simulink model "Controle_controle"  (R2015a)
settings: Solver=ode45  StartTime=0.0  StopTime=Tsim  RelTol=1e-4
undefined symbols (not defined in the file or in its folder): G, sigbuilder_block
settings Model: Creator=pedro  LastModifiedBy=Administrator
settings OptimizationCC: ExpressionDepthLimit=2147483647
settings DebuggingCC: UnderspecifiedInitializationDetection=Classic  MergeDetectMultiDrivingBlocksExec=none  SolverPrmCheckMsg=warning  StateNameClashWarn=warning

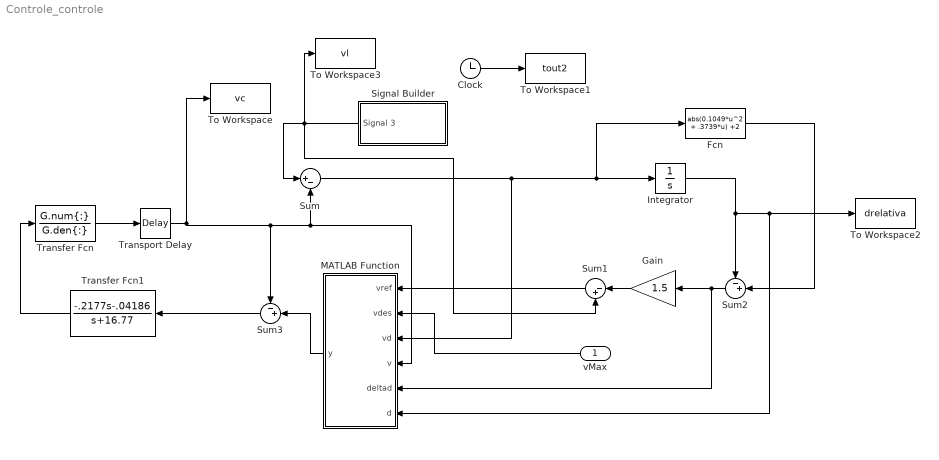
== system Controle_controle ==
  vMax : Inport
  Clock : Clock
  Fcn : Fcn  Expr=abs(0.1049*u^2 + .3739*u) +2
  Gain : Gain  Gain=1.5
  Integrator : Integrator
  MATLAB Function : MATLAB Function  TreatAsAtomicUnit=on
  Signal Builder : Subsystem  Tag=STV Subsys  LoadFcn=sigbuilder_block('load');  StartFcn=sigbuilder_block('start');  StopFcn=sigbuilder_block('stop');  ClipboardFcn=sigbuilder_block('clipboard');  mask(Sigbuilder block){}
      mask help: Simulink:masks:SigbuilderBlock_MD
      mask init:
      | if ~strcmp(get_param(bdroot(gcbh),'SimulationStatus'),'stopped') tuvar = sigbuilder_block('maskInit'); end
      settings: CopyFcn=sigbuilder_block('copy');  DeleteFcn=sigbuilder_block('delete');  ModelCloseFcn=sigbuilder_block('modelClose');  PreSaveFcn=sigbuilder_block('preSave');  PauseFcn=sigbuilder_block('pause');  ContinueFcn=sigbuilder_block('continue');  NameChangeFcn=sigbuilder_block('namechange');  OpenFcn=sigbuilder_block('open',[437.6 199.2 550.4 400 ]);  CloseFcn=sigbuilder_block('close');
      mask Display: plot(0, 0, 100, 100,[2, 2, 32, 32, 2], [68, 8, 8, 68, 68],[32, 2], [38, 38], [32, 19, 2],[53, 60, 44], [32, 17, 17, 2],[16, 16, 31, 31]);txt = getActiveGroup(gcbh);text(2, 100, txt,'verticalAlignment', 'top');
  Sum : Sum  Inputs=|+-
  Sum1 : Sum  Inputs=|-+
  Sum2 : Sum  Inputs=-+|
  Sum3 : Sum  Inputs=-+|
  To Workspace : ToWorkspace  VariableName=vc  SampleTime=-1
  To Workspace1 : ToWorkspace  VariableName=tout2  SampleTime=-1
  To Workspace2 : ToWorkspace  VariableName=drelativa  SampleTime=-1
  To Workspace3 : ToWorkspace  VariableName=vl  SampleTime=-1
  Transfer Fcn : TransferFcn  Numerator=G.num{:}  Denominator=G.den{:}
  Transfer Fcn1 : TransferFcn  Numerator=[-.2177 -.04186]  Denominator=[1 16.77]
  Transport Delay : TransportDelay  DelayTime=G.InputDelay
  wires:
  Integrator/1 -> MATLAB Function/6(d), To Workspace2/1, Sum2/1
  Sum2/1 -> MATLAB Function/5(deltad), Gain/1
  Gain/1 -> Sum1/1
  MATLAB Function/1(y) -> Sum3/2
  Sum1/1 -> MATLAB Function/1(vref)
  Sum/1 -> MATLAB Function/3(vd), Fcn/1, Integrator/1
  vMax/1 -> MATLAB Function/2(vdes)
  Signal Builder/1(Signal 3) -> To Workspace3/1, Sum1/2, Sum/1
  Clock/1 -> To Workspace1/1
  Transfer Fcn/1 -> Transport Delay/1
  Sum3/1 -> Transfer Fcn1/1
  Transfer Fcn1/1 -> Transfer Fcn/1
  Fcn/1 -> Sum2/2
  Transport Delay/1 -> Sum3/1, MATLAB Function/4(v), Sum/2, To Workspace/1

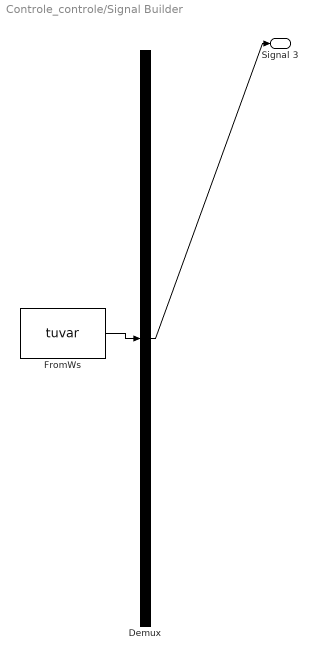
== system Controle_controle/Signal Builder ==
  Demux : Demux  Tag=STV Demux  Outputs=1
  FromWs : FromWorkspace  Tag=STV FromWs  VariableName=tuvar  SampleTime=0
      SigBuilderData=|
      | common.afterFinalStr = 'Extrapolate'
      | common.sampleTime = 0
      | dataSet.timeRange = [0 10000]
      | dataSet.name = 'Group 1'
      | sbobj.Groups.Name = 'Group 1'
      | sbobj.Groups.Signals.Name = 'Signal 3'
      | sbobj.Groups.Signals.XData = [0 2500 5000 7500 10000]
      | sbobj.Groups.Signals.YData = [13.89 13.89 12.5 12.5 14.66]
      | sbobj.Groups.TimeRange = [0 10000]
  Signal 3 : Outport  Tag=STV Outport
  wires:
  FromWs/1 -> Demux/1
  Demux/1 -> Signal 3/1

== matlab function Controle_controle/MATLAB Function ==
  data: vref input; vdes input; y output; vd input; v input; deltad input; d input
function y   = fcn(vref, vdes, vd, v, deltad,d)
%#codegen
%if(deltad<0)
%    y=vdes;
%end

%if(deltad>0 && v<vref)
%    y=vref;
%end


% if(deltad<0)
%     y=vdes;
% elseif(v<vref)
%     y=min(vdes, vref);
% elseif(vd<0)
%     y=min(vdes, vref);
% else
%     y=vdes;
% end

%if(d >=10)

    if(deltad<0)
        y=vdes;
    else
        if(v<vref)
            y=min(vdes, vref);
        else
            if(vd < 0)
                y=min(vdes, vref);
            else
                y = vdes;
            end
        end
    end
% else
%     y = 0;
%     flag = 0;
%end
